simulink model "closedloop"  (R2023b)
settings: Solver=FixedStepAuto  StartTime=0.0  StopTime=5  FixedStep=0.01  RelTol=1e-3
values from neighbouring files (symbols this model uses):
  A = -2    [runsim.m]
  B = 3    [runsim.m]
  C = 1    [runsim.m]
  CA = C*A    (= -2)    [runsim.m]
  D = 0    [runsim.m]
  fc = 1/2    (= 0.5)    [runsim.m]
  invCB = inv(C*B)    [runsim.m]
  K = 4    [runsim.m]
settings Model: Creator=suvo  LastModifiedBy=suvo

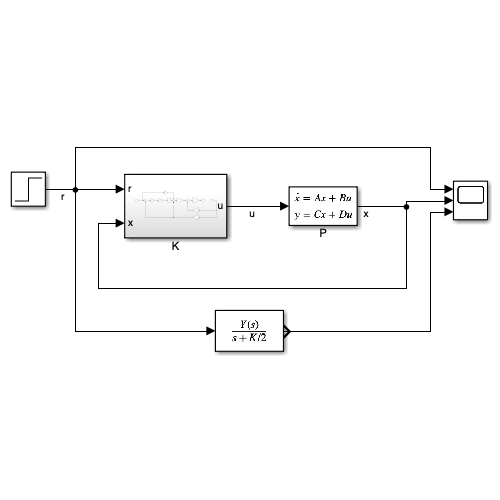
[thumbnail: Simulink's stored preview of the top-level diagram]
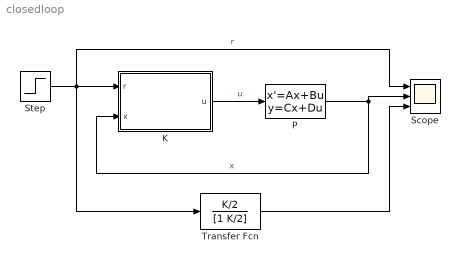
== system closedloop ==
  K : Subsystem
  P : StateSpace  A=A  B=B  C=C  D=D  InitialCondition=0
  Scope : Scope  NumInputPorts=3
  Step : Step  SampleTime=0
  Transfer Fcn : TransferFcn  Numerator=K/2  Denominator=[1 K/2]
  wires:
  K/1(u) -> P/1  "u"
  P/1 -> K/2(x), Scope/2  "x"
  Step/1 -> Transfer Fcn/1, Scope/1, K/1(r)  "r"
  Transfer Fcn/1 -> Scope/3

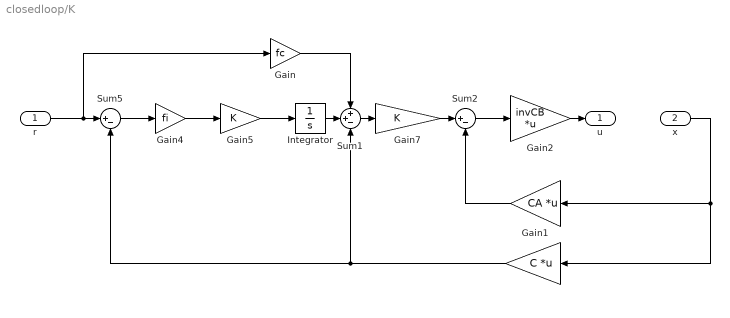
== system closedloop/K ==
  r : Inport
  x : Inport  Port=2
  " " : Gain  Gain=C  Multiplication=Matrix(K*u)
  Gain : Gain  Gain=fc
  Gain1 : Gain  Gain=CA  Multiplication=Matrix(K*u)
  Gain2 : Gain  Gain=invCB  Multiplication=Matrix(K*u)
  Gain4 : Gain  Gain=fi
  Gain5 : Gain  Gain=K
  Gain7 : Gain  Gain=K
  Integrator : Integrator
  Sum1 : Sum  Inputs=++-
  Sum2 : Sum  Inputs=|+-
  Sum5 : Sum  Inputs=|+-
  u : Outport
  wires:
  Gain2/1 -> u/1
  Sum1/1 -> Gain7/1
  r/1 -> Gain/1, Sum5/1
  x/1 -> " "/1, Gain1/1
  Gain5/1 -> Integrator/1
  Sum2/1 -> Gain2/1
  Gain1/1 -> Sum2/2
  Gain/1 -> Sum1/1
  Sum5/1 -> Gain4/1
  Gain4/1 -> Gain5/1
  " "/1 -> Sum5/2, Sum1/3
  Gain7/1 -> Sum2/1
  Integrator/1 -> Sum1/2
